simulink model "filatski_slog"  (Simulink 6.5)
settings: Solver=ode45  StartTime=0.0  StopTime=10.0  RelTol=1e-3
libraries: dsparch4 x4, dspwin32 x2
settings Model: Creator=im41651  LastModifiedBy=im41651  xpc_rtwmakecfg_data=_xpcaudpmc_
settings OptimizationCC: InlineInvariantSignals=on
settings DebuggingCC: MultiTaskDSMMsg=warning  MultiTaskCondExecSysMsg=none  StrictBusMsg=None
settings RTWCC: IncludeERTFirstTime=on

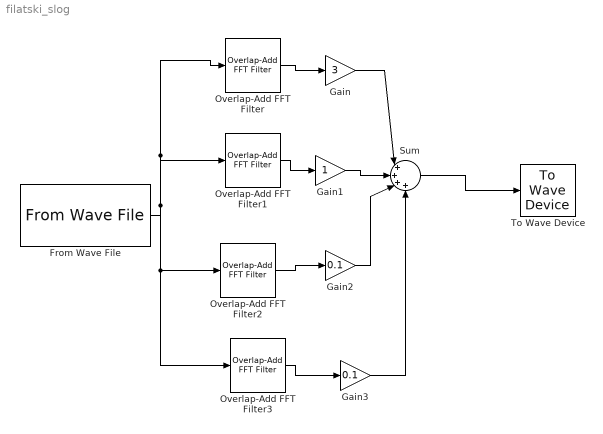
== system filatski_slog ==
  From Wave File : dspwin32/From Wave File  FileName=ivan.wav  SamplesPerFrame=256  MinBufSize=256  dType=double  bLoop=off  timesToPlay=1  restartMode=immediately after last sample  firstSampleOutput=off  lastSampleOutput=off
  Gain : Gain  Gain=3
  Gain1 : Gain
  Gain2 : Gain  Gain=0.1
  Gain3 : Gain  Gain=0.1
  Overlap-Add FFT Filter : dsparch4/Overlap-Add FFT Filter  SystemSampleTime=-1  Nfft=128  h=h1  output_complexity=Real
  Overlap-Add FFT Filter1 : dsparch4/Overlap-Add FFT Filter  SystemSampleTime=-1  Nfft=128  h=h2  output_complexity=Real
  Overlap-Add FFT Filter2 : dsparch4/Overlap-Add FFT Filter  SystemSampleTime=-1  Nfft=128  h=h3  output_complexity=Real
  Overlap-Add FFT Filter3 : dsparch4/Overlap-Add FFT Filter  SystemSampleTime=-1  Nfft=128  h=h4  output_complexity=Real
  Sum : Sum  Inputs=|++++
  To Wave Device : dspwin32/To Wave Device  bufDuration=2  determineBufSize=on  userIntBufSize=256  initDelay=0.1  useDefaultDevice=on  userDeviceID=SigmaTel Audio1  enable24Bit=off
  wires:
  From Wave File/1 -> Overlap-Add FFT Filter/1, Overlap-Add FFT Filter1/1, Overlap-Add FFT Filter2/1, Overlap-Add FFT Filter3/1
  Overlap-Add FFT Filter3/1 -> Gain3/1
  Overlap-Add FFT Filter2/1 -> Gain2/1
  Overlap-Add FFT Filter1/1 -> Gain1/1
  Overlap-Add FFT Filter/1 -> Gain/1
  Gain/1 -> Sum/1
  Gain1/1 -> Sum/2
  Gain2/1 -> Sum/3
  Gain3/1 -> Sum/4
  Sum/1 -> To Wave Device/1
